simulink model "Simple_Moving_Average_Filter"  (R2016a)
settings: Solver=VariableStepAuto  StartTime=0.0  StopTime=100  RelTol=1e-3
undefined symbols (not defined in the file or in its folder): N
libraries: simulink x1, dspstat3 x1, dspindex x1
settings Model: Creator=Cory  LastModifiedBy=Cory

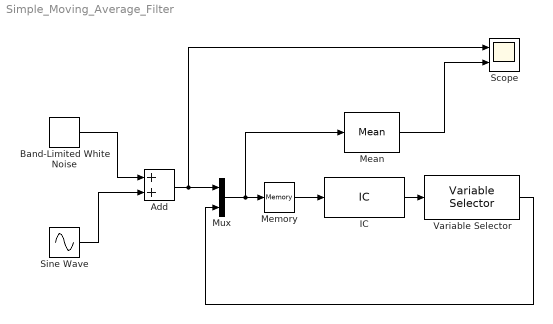
== system Simple_Moving_Average_Filter ==
  Add : Sum
  Band-Limited White Noise : simulink/Sources/Band-Limited White Noise  Cov=[0.1]  Ts=0.1  seed=[23341]
  IC : InitialCondition  Value=[zeros(N,1)]
  Mean : dspstat3/Mean  run=off  reset_popup=None  InputProcessing=Columns as channels (frame based)  directionMode=Each column  dimension=1  roiEnable=off  roiType=Rectangles  roiPortion=Entire ROI  roiOutput=Individual statistics for each ROI  roiFlag=off  outputDataTypeStr=Inherit: Same as accumulator  outputLastDataTypeStr=Inherit: Same as accumulator  outputMin=[]  outputMax=[]  roundingMode=Floor  overflowMode=off
  Memory : Memory
  Mux : Mux  Inputs=2
  Scope : Scope  NumInputPorts=2
  Sine Wave : Sin  Amplitude=10  Frequency=0.1  SampleTime=0
  Variable Selector : dspindex/Variable Selector  NumInputs=1  rowsOrCols=Rows  IdxMode=Fixed  Elements=1:N-1  ZerOneIdxMode=One-based  errmode=Clip Index  FillMode=on  FillValues=0
  wires:
  Band-Limited White Noise/1 -> Add/1
  Sine Wave/1 -> Add/2
  Add/1 -> Scope/1, Mux/1
  Mux/1 -> Mean/1, Memory/1
  Mean/1 -> Scope/2
  Variable Selector/1 -> Mux/2
  IC/1 -> Variable Selector/1
  Memory/1 -> IC/1
